simulink model "speed_to_torque"  (R2018b)
settings: Solver=FixedStepDiscrete  StartTime=0.0  StopTime=4210  FixedStep=sampletime  RelTol=1e-3
values from neighbouring files (symbols this model uses):
  Af = 2.34    [Motor_modell.m]
  alfa = atan(slope/100)    [Motor_modell.m]
  cd = 0.24    [Motor_modell.m]
  fl = 0.88    [Motor_modell.m]
  g = 9.81    [Motor_modell.m]
  k = (0.5334/2)    (= 0.2667)    [Motor_modell.m]
  m = 2108    [Motor_modell.m]
  ro = 1.1846    [Motor_modell.m]
undefined symbols (not defined in the file or in its folder): input, sigbuilder_block
settings Model: Creator=Lac  LastModifiedBy=Lac

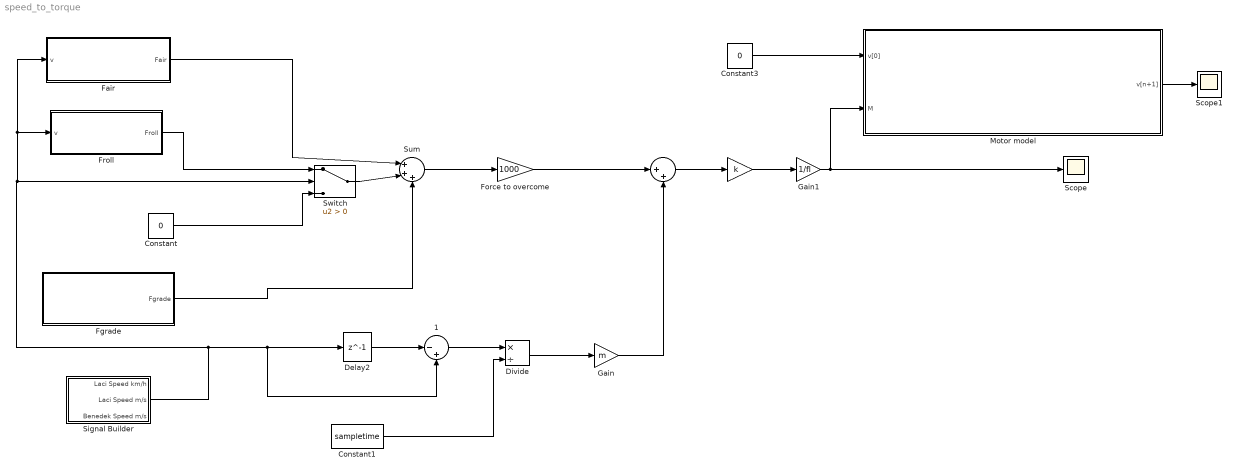
== system speed_to_torque ==
  " " : Gain  Gain=k
  " " : Sum  Inputs=|++
  " 1" : Sum  Inputs=|-+
  Constant : Constant  Value=0
  Constant1 : Constant  Value=sampletime
  Constant3 : Constant  Value=0
  Delay2 : Delay  DelayLength=1  InitialCondition=0
  Divide : Product  Inputs=*/
  "Fair " : Subsystem
  Fgrade : Subsystem
  Force to overcome : Gain  Gain=1000
  Froll : Subsystem
  Gain : Gain  Gain=m
  Gain1 : Gain  Gain=1/fl
  Motor model : Subsystem
      mask Display: image('C:\Users\Lac\Desktop\section-hero-background.jpg');
  Scope : Scope
  Scope1 : Scope
  Signal Builder : Subsystem  Tag=STV Subsys  LoadFcn=sigbuilder_block('load');  StartFcn=sigbuilder_block('start');  StopFcn=sigbuilder_block('stop');  ClipboardFcn=sigbuilder_block('clipboard');  mask(Sigbuilder block){tuvar=[0:10]}
      mask help: Simulink:masks:SigbuilderBlock_MD
      mask init:
      | if ~strcmp(get_param(bdroot(gcbh),'SimulationStatus'),'stopped') tuvar = sigbuilder_block('maskInit'); end
      settings: CopyFcn=sigbuilder_block('copy');  DeleteFcn=sigbuilder_block('delete');  ModelCloseFcn=sigbuilder_block('modelClose');  PreSaveFcn=sigbuilder_block('preSave');  PauseFcn=sigbuilder_block('pause');  ContinueFcn=sigbuilder_block('continue');  NameChangeFcn=sigbuilder_block('namechange');  OpenFcn=sigbuilder_block('open',[5.4 30 1141.2 522.6 ]);  CloseFcn=sigbuilder_block('close');
      mask Display: plot(0, 0, 100, 100,[2, 2, 32, 32, 2], [68, 8, 8, 68, 68],[32, 2], [38, 38], [32, 19, 2],[53, 60, 44], [32, 17, 17, 2],[16, 16, 31, 31]);txt = getActiveGroup(gcbh);text(2, 100, txt,'verticalAlignment', 'top');
  Sum : Sum  Inputs=|+++
  Switch : Switch  Criteria=u2 > Threshold
  wires:
  Divide/1 -> Gain/1
  Switch/1 -> Sum/2
  Sum/1 -> Force to overcome/1
  Constant/1 -> Switch/3
  Constant3/1 -> Motor model/1(v[0])
  Motor model/1(v[n+1]) -> Scope1/1
  Gain/1 -> " "/2
  " "/1 -> Gain1/1
  Signal Builder/2(Laci Speed m/s) -> Delay2/1, " 1"/2, "Fair "/1(v), Froll/1(v), Switch/2
  Force to overcome/1 -> " "/1
  " "/1 -> " "/1
  Gain1/1 -> Motor model/2("M "), Scope/1
  Froll/1(Froll) -> Switch/1
  "Fair "/1(Fair) -> Sum/1
  Fgrade/1(Fgrade) -> Sum/3
  Delay2/1 -> " 1"/1
  " 1"/1 -> Divide/1
  Constant1/1 -> Divide/2

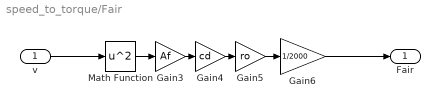
== system speed_to_torque/Fair  ==
  v : Inport
  Gain3 : Gain  Gain=Af
  Gain4 : Gain  Gain=cd
  Gain5 : Gain  Gain=ro
  Gain6 : Gain  Gain=1/2000
  Math Function : Math  Operator=square  SaturateOnIntegerOverflow=on
  Fair : Outport
  wires:
  Math Function/1 -> Gain3/1
  Gain4/1 -> Gain5/1
  Gain3/1 -> Gain4/1
  Gain5/1 -> Gain6/1
  v/1 -> Math Function/1
  Gain6/1 -> Fair/1

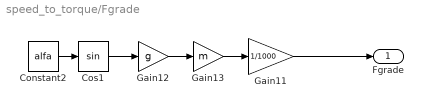
== system speed_to_torque/Fgrade ==
  Constant2 : Constant  Value=alfa
  Cos1 : Trigonometry
  Gain11 : Gain  Gain=1/1000
  Gain12 : Gain  Gain=g
  Gain13 : Gain  Gain=m
  Fgrade : Outport
  wires:
  Gain13/1 -> Gain11/1
  Constant2/1 -> Cos1/1
  Cos1/1 -> Gain12/1
  Gain12/1 -> Gain13/1
  Gain11/1 -> Fgrade/1

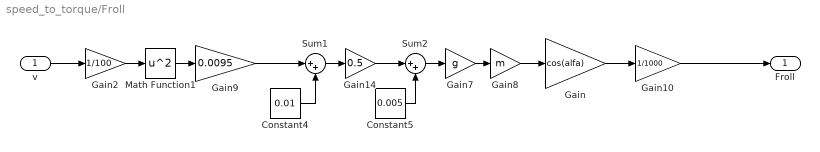
== system speed_to_torque/Froll ==
  v : Inport
  Constant4 : Constant  Value=0.01
  Constant5 : Constant  Value=0.005
  Gain : Gain  Gain=cos(alfa)
  Gain10 : Gain  Gain=1/1000
  Gain14 : Gain  Gain=0.5
  Gain2 : Gain  Gain=1/100
  Gain7 : Gain  Gain=g
  Gain8 : Gain  Gain=m
  Gain9 : Gain  Gain=0.0095
  Math Function1 : Math  Operator=square  SaturateOnIntegerOverflow=on
  Sum1 : Sum  Inputs=|++
  Sum2 : Sum  Inputs=|++
  Froll : Outport
  wires:
  Gain8/1 -> Gain/1
  Constant4/1 -> Sum1/2
  Sum2/1 -> Gain7/1
  Gain9/1 -> Sum1/1
  Sum1/1 -> Gain14/1
  Gain10/1 -> Froll/1
  Constant5/1 -> Sum2/2
  Math Function1/1 -> Gain9/1
  Gain14/1 -> Sum2/1
  Gain7/1 -> Gain8/1
  Gain2/1 -> Math Function1/1
  v/1 -> Gain2/1
  Gain/1 -> Gain10/1

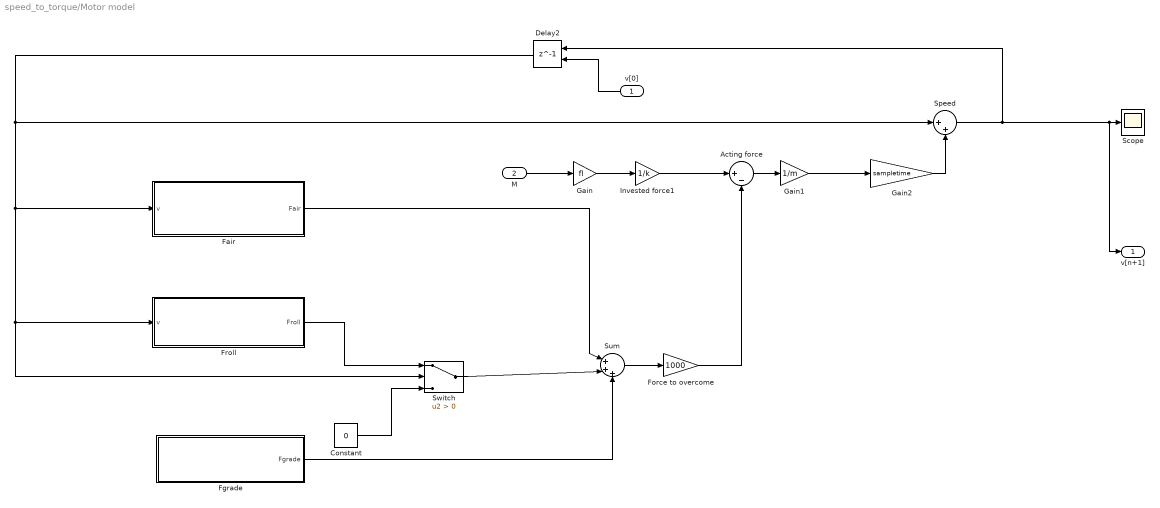
== system speed_to_torque/Motor model ==
  v[0] : Inport
  "M " : Inport  Port=2
  "Acting force " : Sum  Inputs=|+-
  Constant : Constant  Value=0
  Delay2 : Delay  DelayLength=1  InitialConditionSource=Input port  InitialCondition=input
      settings: InputPortMap=u0,p4
  "Fair " : Subsystem
  Fgrade : Subsystem
  Force to overcome : Gain  Gain=1000
  Froll : Subsystem
  Gain : Gain  Gain=fl
  Gain1 : Gain  Gain=1/m
  Gain2 : Gain  Gain=sampletime
  Invested force1 : Gain  Gain=1/k
  Scope : Scope
  "Speed " : Sum  Inputs=|++
  Sum : Sum  Inputs=|+++
  Switch : Switch  Criteria=u2 > Threshold
  v[n+1] : Outport
  wires:
  Delay2/1 -> Switch/2, Froll/1(v), "Fair "/1(v), "Speed "/1
  Invested force1/1 -> "Acting force "/1
  Force to overcome/1 -> "Acting force "/2
  Constant/1 -> Switch/3
  Switch/1 -> Sum/2
  "Speed "/1 -> v[n+1]/1, Scope/1, Delay2/1
  Gain1/1 -> Gain2/1
  Sum/1 -> Force to overcome/1
  Gain2/1 -> "Speed "/2
  Fgrade/1(Fgrade) -> Sum/3
  "Fair "/1(Fair) -> Sum/1
  "Acting force "/1 -> Gain1/1
  v[0]/1 -> Delay2/2
  "M "/1 -> Gain/1
  Gain/1 -> Invested force1/1
  Froll/1(Froll) -> Switch/1

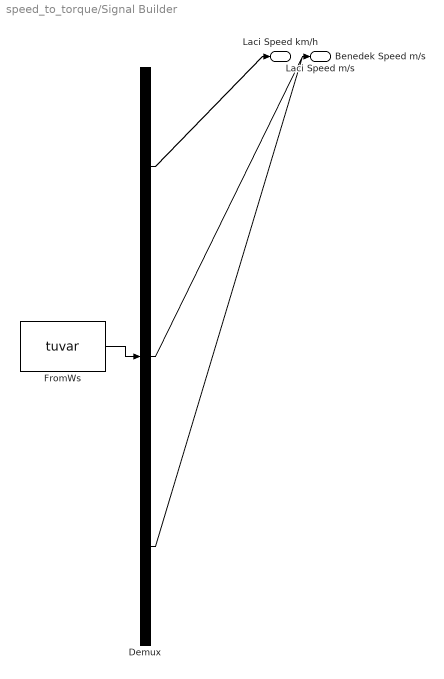
== system speed_to_torque/Signal Builder ==
  Demux : Demux  Tag=STV Demux  Outputs=3
  FromWs : FromWorkspace  Tag=STV FromWs  VariableName=tuvar  SampleTime=0
      SigBuilderData=|
      | common.afterFinalStr = 'Extrapolate'
      | common.sampleTime = 0
      | dataSet.timeRange = [0 7818]
      | dataSet.name = 'Group 1'
      | sbobj.Groups.Name = 'Group 1'
      | sbobj.Groups.Signals(1).Name = 'Laci Speed km/h'
      | sbobj.Groups.Signals(1).XData = [0 5 10 15 20 25 30 35 40 45 50 55 ... (483 elements, 1x483)]
      | sbobj.Groups.Signals(1).YData = [0 30 30 30 30 30 30 30 30 30 30 30 30 30 30 30 30 30 30 30 30 30 30 30 30 30 30 30 30 30 30 30 30 30 30 30 30 30 30 30 30 50 50 50 50 50 50 50 50 50 50 50 50 50 50 50 50 50 50 50 50 50 50 50 50 50 50 50 50 90 90 90 90 90 90 90 90 90 90 90 90 90 90 90 90 90 90 90 50 50 50 50 50 50 50 50 50 50 50 50 50 50 50 50 50 50 50 50 50 50 50 50 50 50 50 50 50 50 50 50 50 50 50 50 0 0 0 0 50 50 50 50 50 50 50 50 50 50 50 50 50 50 50 50 50 50 50 50 50 50 50 50 50 50 50 50 50 50 50 50 50 50 50 50 50 50 50 50 50 50 50 50 50 50 50 50 50 50 50 50 50 50 50 50 50 50 50 50 50 50 50 50 50 50 50 50 50 50 50 50 50 50 50 50 50 50 50 50 50 50 60 60 60 60 60 0 0 0 0 60 60 0 0 0 0 60 60 60 60 0 0 0 0 60 60 60 0 0 0 0 60 60 60 60 60 60 60 60 60 60 60 60 60 60 60 60 0 0 0 0 50 50 0 0 0 0 50 50 50 50 50 50 0 0 0 0 50 50 50 50 0 0 0 0 50 50 50 0 0 0 0 50 50 50 0 0 0 0 50 50 0 0 0 0 50 50 50 50 50 50 0 0 0 0 50 50 0 0 0 0 50 50 50 0 0 0 0 50 50 0 0 0 0 50 50 50 50 50 50 50 50 50 50 0 0 0 0 50 50 50 50 50 50 0 0 0 0 50 50 50 50 50 0 0 0 0 50 50 50 0 0 0 0 50 50 50 0 0 0 0 50 50 50 50 50 0 0 0 0 50 0 0 0 0 50 50 50 0 0 0 0 50 50 50 0 0 0 50 50 50 50 50 0 0 0 0 50 50 50 50 0 0 0 0 50 50 0 0 0 40 40 40 40 70 70 70 70 70 70 70 50 50 50 0 0 0 0 50 50 0 0 0 0 50 50 50 50 50 50 70 70 70 70 70 70 70 60 60 60 60 60 60 50 50 0 0 0 0 50 50 50 50 50]
      | sbobj.Groups.Signals(2).Name = 'Laci Speed m/s'
      | sbobj.Groups.Signals(2).XData = [0 5 10 15 20 25 30 35 40 45 50 55 ... (483 elements, 1x483)]
      | sbobj.Groups.Signals(2).YData = [0 8.33333333333 8.33333333333 8.33333333333 8.33333333333 8.33333333333 8.33333333333 8.33333333333 8.33333333333 8.33333333333 8.33333333333 8.33333333333 ... (483 elements, 1x483)]
      | sbobj.Groups.Signals(3).Name = 'Benedek Speed m/s'
      | sbobj.Groups.Signals(3).XData = [0 1 2 3 4 5 6 7 8 9 10 11 ... (7819 elements, 1x7819)]
      | sbobj.Groups.Signals(3).YData = [2.77777777778 2.77777777778 2.77777777778 2.77777777778 2.77777777778 2.77777777778 2.77777777778 2.77777777778 2.77777777778 2.77777777778 2.77777777778 2.77777777778 ... (7819 elements, 1x7819)]
      | sbobj.Groups.TimeRange = [0 7818]
  Laci Speed km/h : Outport  Tag=STV Outport
  Laci Speed m/s : Outport  Tag=STV Outport  Port=2
  Benedek Speed m/s : Outport  Tag=STV Outport  Port=3
  wires:
  FromWs/1 -> Demux/1
  Demux/1 -> Laci Speed km/h/1
  Demux/2 -> Laci Speed m/s/1
  Demux/3 -> Benedek Speed m/s/1

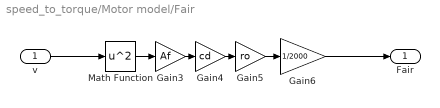
== system speed_to_torque/Motor model/Fair  ==
  v : Inport
  Gain3 : Gain  Gain=Af
  Gain4 : Gain  Gain=cd
  Gain5 : Gain  Gain=ro
  Gain6 : Gain  Gain=1/2000
  Math Function : Math  Operator=square  SaturateOnIntegerOverflow=on
  Fair : Outport
  wires:
  Math Function/1 -> Gain3/1
  Gain4/1 -> Gain5/1
  Gain3/1 -> Gain4/1
  Gain5/1 -> Gain6/1
  v/1 -> Math Function/1
  Gain6/1 -> Fair/1

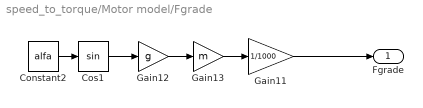
== system speed_to_torque/Motor model/Fgrade ==
  Constant2 : Constant  Value=alfa
  Cos1 : Trigonometry
  Gain11 : Gain  Gain=1/1000
  Gain12 : Gain  Gain=g
  Gain13 : Gain  Gain=m
  Fgrade : Outport
  wires:
  Gain13/1 -> Gain11/1
  Constant2/1 -> Cos1/1
  Cos1/1 -> Gain12/1
  Gain12/1 -> Gain13/1
  Gain11/1 -> Fgrade/1

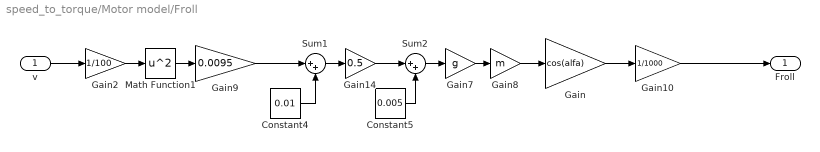
== system speed_to_torque/Motor model/Froll ==
  v : Inport
  Constant4 : Constant  Value=0.01
  Constant5 : Constant  Value=0.005
  Gain : Gain  Gain=cos(alfa)
  Gain10 : Gain  Gain=1/1000
  Gain14 : Gain  Gain=0.5
  Gain2 : Gain  Gain=1/100
  Gain7 : Gain  Gain=g
  Gain8 : Gain  Gain=m
  Gain9 : Gain  Gain=0.0095
  Math Function1 : Math  Operator=square  SaturateOnIntegerOverflow=on
  Sum1 : Sum  Inputs=|++
  Sum2 : Sum  Inputs=|++
  Froll : Outport
  wires:
  Gain8/1 -> Gain/1
  Constant4/1 -> Sum1/2
  Sum2/1 -> Gain7/1
  Gain9/1 -> Sum1/1
  Sum1/1 -> Gain14/1
  Gain10/1 -> Froll/1
  Constant5/1 -> Sum2/2
  Math Function1/1 -> Gain9/1
  Gain14/1 -> Sum2/1
  Gain7/1 -> Gain8/1
  Gain2/1 -> Math Function1/1
  v/1 -> Gain2/1
  Gain/1 -> Gain10/1
